simulink model "IEEE9_16b_1"  (R2020a)
settings: Solver=ode15s  StartTime=0.0  StopTime=5  MaxStep=1e-4  RelTol=1e-3
undefined symbols (not defined in the file or in its folder): k
libraries: powerlib_meascontrol x29, powerlib x27, simulink_extras x26, sps_avr x3
(part 2 of 2)

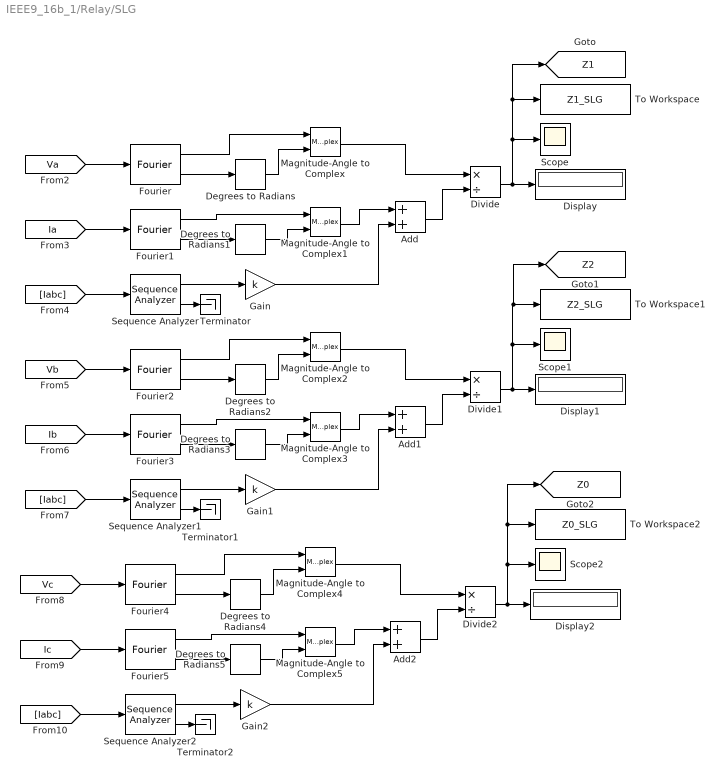
== system IEEE9_16b_1/Relay/SLG ==
  Add : Sum
  Add1 : Sum
  Add2 : Sum
  Degrees to Radians{,1..5} (6 alike) : simulink_extras/Transformations/Degrees to Radians
  Display : Display
  Display1 : Display
  Display2 : Display
  Divide : Product  Inputs=*/
  Divide1 : Product  Inputs=*/
  Divide2 : Product  Inputs=*/
  Fourier{,1..5} (6 alike) : powerlib_meascontrol/Measurements/Fourier  Freq=60  n=1  InInit=[0, 0]  Ts=0
  Gain : Gain  Gain=k
  Gain1 : Gain  Gain=k
  Gain2 : Gain  Gain=k
  Magnitude-Angle to Complex{,1..5} (6 alike) : MagnitudeAngleToComplex
  Scope : Scope
  Scope1 : Scope
  Scope2 : Scope
  Sequence Analyzer : powerlib_meascontrol/Measurements/Sequence Analyzer  Freq=60  n=1  seq=Zero  InInit=[1, 0]  Ts=0
      settings: SourceProductBaseCode=PS
  Sequence Analyzer1 : powerlib_meascontrol/Measurements/Sequence Analyzer  Freq=60  n=1  seq=Zero  InInit=[1, 0]  Ts=0
      settings: SourceProductBaseCode=PS
  Sequence Analyzer2 : powerlib_meascontrol/Measurements/Sequence Analyzer  Freq=60  n=1  seq=Zero  InInit=[1, 0]  Ts=0
      settings: SourceProductBaseCode=PS
  Terminator : Terminator
  Terminator1 : Terminator
  Terminator2 : Terminator
  To Workspace : ToWorkspace  VariableName=Z1_SLG  SaveFormat=Timeseries  SampleTime=-1
  To Workspace1 : ToWorkspace  VariableName=Z2_SLG  SaveFormat=Timeseries  SampleTime=-1
  To Workspace2 : ToWorkspace  VariableName=Z0_SLG  SaveFormat=Timeseries  SampleTime=-1
  tag scope: Z0=global, Z1=global, Z2=global
  wires:
  Gain/1 -> Add/2
  Gain1/1 -> Add1/2
  Magnitude-Angle to Complex3/1 -> Add1/1
  Fourier1/2 -> Degrees to Radians1/1
  Sequence Analyzer1/1 -> Gain1/1
  [Va] -> Fourier/1
  Sequence Analyzer2/1 -> Gain2/1
  Magnitude-Angle to Complex/1 -> Divide/1
  Fourier1/1 -> Magnitude-Angle to Complex1/1
  Degrees to Radians/1 -> Magnitude-Angle to Complex/2
  Add/1 -> Divide/2
  Sequence Analyzer/1 -> Gain/1
  [Ib] -> Fourier3/1
  Fourier3/2 -> Degrees to Radians3/1
  Add1/1 -> Divide1/2
  Divide2/1 -> [Z0], To Workspace2/1, Scope2/1, Display2/1
  Fourier/1 -> Magnitude-Angle to Complex/1
  [Iabc] -> Sequence Analyzer/1
  Add2/1 -> Divide2/2
  Fourier4/2 -> Degrees to Radians4/1
  Magnitude-Angle to Complex1/1 -> Add/1
  Fourier/2 -> Degrees to Radians/1
  Degrees to Radians5/1 -> Magnitude-Angle to Complex5/2
  Degrees to Radians1/1 -> Magnitude-Angle to Complex1/2
  [Ia] -> Fourier1/1
  Divide1/1 -> Display1/1, Scope1/1, [Z2], To Workspace1/1
  Divide/1 -> [Z1], To Workspace/1, Scope/1, Display/1
  Degrees to Radians3/1 -> Magnitude-Angle to Complex3/2
  Magnitude-Angle to Complex2/1 -> Divide1/1
  Fourier4/1 -> Magnitude-Angle to Complex4/1
  [Vc] -> Fourier4/1
  Sequence Analyzer1/2 -> Terminator1/1
  Degrees to Radians2/1 -> Magnitude-Angle to Complex2/2
  Sequence Analyzer2/2 -> Terminator2/1
  Fourier3/1 -> Magnitude-Angle to Complex3/1
  Gain2/1 -> Add2/2
  [Ic] -> Fourier5/1
  Fourier2/1 -> Magnitude-Angle to Complex2/1
  Degrees to Radians4/1 -> Magnitude-Angle to Complex4/2
  Magnitude-Angle to Complex5/1 -> Add2/1
  [Iabc] -> Sequence Analyzer1/1
  [Vb] -> Fourier2/1
  Fourier2/2 -> Degrees to Radians2/1
  Sequence Analyzer/2 -> Terminator/1
  Fourier5/1 -> Magnitude-Angle to Complex5/1
  Fourier5/2 -> Degrees to Radians5/1
  Magnitude-Angle to Complex4/1 -> Divide2/1
  [Iabc] -> Sequence Analyzer2/1

== matlab function IEEE9_16b_1/Relay/MATLAB Function ==
  settings: updateMethod=DISCRETE
  data: Vabc input; Za output; Iabc input; Zb output; Zc output; Zab output; Zbc output; Zca output; Za_3ph output; Zb_3ph output; Zc_3ph output; T1 output; T2 output; T3 output
function [Za, Zb, Zc, Zab, Zbc, Zca, Za_3ph, Zb_3ph, Zc_3ph, T1, T2, T3] = fcn(Vabc, Iabc)
 
persistent init C1 C2 C3 r1 r2 r3 trip1 trip2 trip3 k
if isempty(init)  
    trip1 = false; trip2 = false; trip3 = false;
    Zline = 100*(0.0449 + 1i*2*pi*60*1.01e-3);
    Z0_line = 100*(0.11241 + 1i*60*2.02e-3*2*pi);
    k = (Z0_line - Zline)./Zline;
    Z1 = 0.80*Zline;
    Z2 = 1.2*Zline;
    Z3 = 2*abs(Zline)*exp(1i*80*pi/180);
    C1 = Z1/2; C2 = Z2/2; C3 = Z3/2;
    r1 = abs(C1); r2 = abs(C2); r3 = abs(C3);
    MTA1 = angle(Z1);
    MTA2 = angle(Z2);
    MTA3 = 80*pi/180;
    init = 1;
    
%     circle(real(C1),imag(C1),r1)
%     circle(real(C2),imag(C2),r2)
%     circle(real(C3),imag(C3),r3)
end

Va = Vabc(1); Vb = Vabc(2); Vc = Vabc(3);
Ia = Iabc(1); Ib = Iabc(2); Ic =Iabc(3);
Io = (Ia+Ib+Ic)/3;

Za = Va/(Ia+k*Io);
Zb = Vb/(Ib+k*Io);
Zc = Vc/(Ic+k*Io);
Zab = (Va-Vb)/(Ia-Ib);
Zbc = (Vb-Vc)/(Ib-Ic);
Zca = (Vc-Va)/(Ic-Ia);
Za_3ph = Va/Ia;
Zb_3ph = Vb/Ib;
Zc_3ph = Vc/Ic;

if any([abs(Za-C1),abs(Zb-C1),abs(Zc-C1),abs(Zab-C1),abs(Zbc-C1),abs(Zca-C1),abs(Za_3ph-C1),abs(Zb_3ph-C1),abs(Zc_3ph-C1)] <= r1)
    trip1 = true;
elseif any([abs(Za-C2),abs(Zb-C2),abs(Zc-C2),abs(Zab-C2),abs(Zbc-C2),abs(Zca-C2),abs(Za_3ph-C2),abs(Zb_3ph-C2),abs(Zc_3ph-C2)] <= r2)
    trip2 = true;
elseif any([abs(Za-C3),abs(Zb-C3),abs(Zc-C3),abs(Zab-C3),abs(Zbc-C3),abs(Zca-C3),abs(Za_3ph-C3),abs(Zb_3ph-C3),abs(Zc_3ph-C3)] <= r3)
    trip3 = true;
end

T1 =trip1; T2 = trip2; T3 = trip3;
end
